simulink model "FIR_Filter"  (R2020a)
settings: Solver=FixedStepAuto  StartTime=0.0  StopTime=10.0  FixedStep=0.2  RelTol=1e-3
settings Model: Creator=Hp  LastModifiedBy=Hp
settings DataIOCC: SaveOutput=off  SaveTime=off

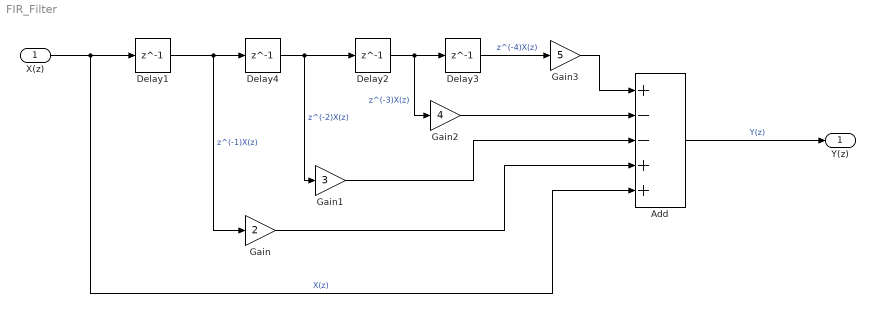
== system FIR_Filter ==
  X(z) : Inport  OutDataTypeStr=double  PortDimensions=1  SampleTime=[0.20000000000000001,0]
  Add : Sum  Inputs=+--++
  Delay{1..4} (4 alike) : Delay  DelayLength=1
  Gain : Gain  Gain=2
  Gain1 : Gain  Gain=3
  Gain2 : Gain  Gain=4
  Gain3 : Gain  Gain=5
  Y(z) : Outport  OutDataTypeStr=double  PortDimensions=1  SampleTime=[0.20000000000000001,0]
  wires:
  Gain/1 -> Add/4
  Gain2/1 -> Add/2
  Gain3/1 -> Add/1
  X(z)/1 -> Add/5, Delay1/1  "X(z)"
  Delay3/1 -> Gain3/1  "z^(-4)X(z)"
  Delay2/1 -> Gain2/1, Delay3/1  "z^(-3)X(z)"
  Delay4/1 -> Gain1/1, Delay2/1  "z^(-2)X(z)"
  Delay1/1 -> Delay4/1, Gain/1  "z^(-1)X(z)"
  Gain1/1 -> Add/3
  Add/1 -> Y(z)/1  "Y(z)"
